simulink model "Antriebsstrangmodell_V1_4_n5_WHasym"  (R2019a)
settings: Solver=FixedStepAuto  StartTime=0.0  StopTime=t_Simulation  FixedStep=dt  RelTol=1e-3
values from neighbouring files (symbols this model uses):
  A_Stirn = 2    [Simulation_Antriebsstrangmodell_V1_4_n5_WHasym.m]    (also in Simulation_Antriebsstrangmodell_V1_4_n5_WHasym_S1.m)
  alpha_Luft = -4e-3    (= -0.004)    [Simulation_Antriebsstrangmodell_V1_4_n5_WHasym.m]    (also in Simulation_Antriebsstrangmodell_V1_4_n5_WHasym_S1.m)
  alpha_Rotor = alpha_Al    (= 0.004)    [Simulation_Antriebsstrangmodell_V1_4_n5_WHasym.m]    (also in Simulation_Antriebsstrangmodell_V1_4_n5_WHasym_S1.m)
  alpha_Stator = alpha_Al    (= 0.004)    [Simulation_Antriebsstrangmodell_V1_4_n5_WHasym.m]    (also in Simulation_Antriebsstrangmodell_V1_4_n5_WHasym_S1.m)
  alpha_Ummag = -0.75e-3    (= -0.00075)    [Simulation_Antriebsstrangmodell_V1_4_n5_WHasym.m]    (also in Simulation_Antriebsstrangmodell_V1_4_n5_WHasym_S1.m)
  c_W = 0.37    [Simulation_Antriebsstrangmodell_V1_4_n5_WHasym.m]    (also in Simulation_Antriebsstrangmodell_V1_4_n5_WHasym_S1.m)
  cp_Luft = 1008.8    [Simulation_Antriebsstrangmodell_V1_4_n5_WHasym.m]    (also in Simulation_Antriebsstrangmodell_V1_4_n5_WHasym_S1.m)
  e_Fahrzeug = 1.0478    [Simulation_Antriebsstrangmodell_V1_4_n5_WHasym.m]    (also in Simulation_Antriebsstrangmodell_V1_4_n5_WHasym_S1.m)
  eta_EMaschine_Break_M_EMaschine = flipud(KennfeldMaschine.M(:,1))'    [Simulation_Antriebsstrangmodell_V1_4_n5_WHasym.m]    (also in Simulation_Antriebsstrangmodell_V1_4_n5_WHasym_S1.m)
  eta_EMaschine_Break_M_EMaschine_reku = -KennfeldMaschine.M(:,1)'    [Simulation_Antriebsstrangmodell_V1_4_n5_WHasym.m]    (also in Simulation_Antriebsstrangmodell_V1_4_n5_WHasym_S1.m)
  eta_EMaschine_Break_n_EMaschine = KennfeldMaschine.n(end-1,:)    [Simulation_Antriebsstrangmodell_V1_4_n5_WHasym.m]    (also in Simulation_Antriebsstrangmodell_V1_4_n5_WHasym_S1.m)
  eta_EMaschine_Break_n_EMaschine_reku = KennfeldMaschine.n(end-1,:)    [Simulation_Antriebsstrangmodell_V1_4_n5_WHasym.m]    (also in Simulation_Antriebsstrangmodell_V1_4_n5_WHasym_S1.m)
  eta_EMaschine_Faktor_Volllast = 0.98    [Simulation_Antriebsstrangmodell_V1_4_n5_WHasym.m]    (also in Simulation_Antriebsstrangmodell_V1_4_n5_WHasym_S1.m)
  eta_EMaschine_Table = flip(KennfeldMaschine.etages,1)    [Simulation_Antriebsstrangmodell_V1_4_n5_WHasym.m]    (also in Simulation_Antriebsstrangmodell_V1_4_n5_WHasym_S1.m)
  eta_EMaschine_Table_reku = KennfeldMaschine.etages    [Simulation_Antriebsstrangmodell_V1_4_n5_WHasym.m]    (also in Simulation_Antriebsstrangmodell_V1_4_n5_WHasym_S1.m)
  eta_Getriebe = 0.96    [Simulation_Antriebsstrangmodell_V1_4_n5_WHasym.m]    (also in Simulation_Antriebsstrangmodell_V1_4_n5_WHasym_S1.m)
  eta_IA = 0.5    [Simulation_Antriebsstrangmodell_V1_4_n5_WHasym.m]    (also in Simulation_Antriebsstrangmodell_V1_4_n5_WHasym_S1.m)
  h_WC_pumpoff = Nu_WC*lam_WC/dh_WC    [Simulation_Antriebsstrangmodell_V1_4_n5_WHasym.m]    (also in Simulation_Antriebsstrangmodell_V1_4_n5_WHasym_S1.m)
  h_WC_pumpon = Nu_WC*lam_WC/dh_WC    [Simulation_Antriebsstrangmodell_V1_4_n5_WHasym.m]    (also in Simulation_Antriebsstrangmodell_V1_4_n5_WHasym_S1.m)
  i_Getriebe = 5.697    [Simulation_Antriebsstrangmodell_V1_4_n5_WHasym.m]    (also in Simulation_Antriebsstrangmodell_V1_4_n5_WHasym_S1.m)
  krb_Korrektur = 0.53/10    (= 0.053)    [Simulation_Antriebsstrangmodell_V1_4_n5_WHasym.m]    (also in Simulation_Antriebsstrangmodell_V1_4_n5_WHasym_S1.m)
  lam_Luft = 0.028592    [Simulation_Antriebsstrangmodell_V1_4_n5_WHasym.m]    (also in Simulation_Antriebsstrangmodell_V1_4_n5_WHasym_S1.m)
  M_EMaschine_max = zeros(2,numel(eta_EMaschine_Break_n_EMaschine))    [Simulation_Antriebsstrangmodell_V1_4_n5_WHasym.m]    (also in Simulation_Antriebsstrangmodell_V1_4_n5_WHasym_S1.m)
  m_Fahrzeug = 825    [Simulation_Antriebsstrangmodell_V1_4_n5_WHasym.m]    (also in Simulation_Antriebsstrangmodell_V1_4_n5_WHasym_S1.m)
  m_Zuladung = 80    [Simulation_Antriebsstrangmodell_V1_4_n5_WHasym.m]    (also in Simulation_Antriebsstrangmodell_V1_4_n5_WHasym_S1.m)
  nue_Luft = 19.230034390524e-6    (= 1.92300343905e-05)    [Simulation_Antriebsstrangmodell_V1_4_n5_WHasym.m]    (also in Simulation_Antriebsstrangmodell_V1_4_n5_WHasym_S1.m)
  pump_start_limit = 273.15 + 33    (= 306.15)    [Simulation_Antriebsstrangmodell_V1_4_n5_WHasym.m]    (also in Simulation_Antriebsstrangmodell_V1_4_n5_WHasym_S1.m)
  r_dynamisch = 0.2774    [Simulation_Antriebsstrangmodell_V1_4_n5_WHasym.m]    (also in Simulation_Antriebsstrangmodell_V1_4_n5_WHasym_S1.m)
  rho_Luft = 1.2    [Simulation_Antriebsstrangmodell_V1_4_n5_WHasym.m]    (also in Simulation_Antriebsstrangmodell_V1_4_n5_WHasym_S1.m)
  rho_Luft_EM = 1.0468    [Simulation_Antriebsstrangmodell_V1_4_n5_WHasym.m]    (also in Simulation_Antriebsstrangmodell_V1_4_n5_WHasym_S1.m)
  share_EMaschine_Ummagnet_reku_Table = ser.gen.share_Ummagnetisierungsverluste    [Simulation_Antriebsstrangmodell_V1_4_n5_WHasym.m]    (also in Simulation_Antriebsstrangmodell_V1_4_n5_WHasym_S1.m)
  share_EMaschine_Ummagnet_Table = ser.mot.share_Ummagnetisierungsverluste    [Simulation_Antriebsstrangmodell_V1_4_n5_WHasym.m]    (also in Simulation_Antriebsstrangmodell_V1_4_n5_WHasym_S1.m)
  share_EMaschine_Wicklung_reku_Table = ser.gen.share_Wicklungsverluste    [Simulation_Antriebsstrangmodell_V1_4_n5_WHasym.m]    (also in Simulation_Antriebsstrangmodell_V1_4_n5_WHasym_S1.m)
  share_EMaschine_Wicklung_Table = ser.mot.share_Wicklungsverluste    [Simulation_Antriebsstrangmodell_V1_4_n5_WHasym.m]    (also in Simulation_Antriebsstrangmodell_V1_4_n5_WHasym_S1.m)
  share_EMaschine_WirkMech_reku_Table = ser.gen.share_WirkmechVerluste    [Simulation_Antriebsstrangmodell_V1_4_n5_WHasym.m]    (also in Simulation_Antriebsstrangmodell_V1_4_n5_WHasym_S1.m)
  share_EMaschine_WirkMech_Table = ser.mot.share_WirkmechVerluste    [Simulation_Antriebsstrangmodell_V1_4_n5_WHasym.m]    (also in Simulation_Antriebsstrangmodell_V1_4_n5_WHasym_S1.m)
  share_EMaschine_WirkZus_reku_Table = ser.gen.share_WirkZusVerl    [Simulation_Antriebsstrangmodell_V1_4_n5_WHasym.m]    (also in Simulation_Antriebsstrangmodell_V1_4_n5_WHasym_S1.m)
  share_EMaschine_WirkZus_Table = ser.mot.share_WirkZusVerl    [Simulation_Antriebsstrangmodell_V1_4_n5_WHasym.m]    (also in Simulation_Antriebsstrangmodell_V1_4_n5_WHasym_S1.m)
  T_Entwurf_Rotor = 273.15+20    (= 293.15)    [Simulation_Antriebsstrangmodell_V1_4_n5_WHasym.m]    (also in Simulation_Antriebsstrangmodell_V1_4_n5_WHasym_S1.m)
  T_Entwurf_Stator = 273.15+20    (= 293.15)    [Simulation_Antriebsstrangmodell_V1_4_n5_WHasym.m]    (also in Simulation_Antriebsstrangmodell_V1_4_n5_WHasym_S1.m)
  t_Simulation = v_Fahrzeug.Time(end)+1    [Simulation_Antriebsstrangmodell_V1_4_n5_WHasym.m]    (also in Simulation_Antriebsstrangmodell_V1_4_n5_WHasym_S1.m = v_Fahrzeug.Time(end))
  T_Start_EMaschine = 273.15 + 23    (= 296.15)    [Simulation_Antriebsstrangmodell_V1_4_n5_WHasym.m]    (also in Simulation_Antriebsstrangmodell_V1_4_n5_WHasym_S1.m)
  v_max = 110    [Simulation_Antriebsstrangmodell_V1_4_n5_WHasym.m]    (also in Simulation_Antriebsstrangmodell_V1_4_n5_WHasym_S1.m)
undefined symbols (not defined in the file or in its folder): A_AGP, A_IA, Anteil_Rotor_Ringe, Anteil_Stator, chi_Lager, D_2a, D_2r, delta, f_R, m_RTO, m_RYO, m_SSL_L, m_STO, m_SYO, m_WH1_L, m_WH2_L, n_dis
libraries: fl_lib x440, nesl_utility x106, SimscapeCustomBlocks_lib x45, simulink x3
(part 5 of 5)

== system Antriebsstrangmodell_V1_4_n5_WHasym/Antriebsstrang/E-Maschine Thermik/Wärmeübergangskoeffizienten Konvektion Luftspalt und Endcap-Luft/Endcap-Luft-Konvektion ==
  note: HTC_fconv stellt den Wärmeübergangs-
      | koeffizienten der erzwungen dar. Für diesen
      | wird bloß der geschwindigkeitsabhängige
      | Teil der empirischen Konvektions-Korrelation
      | der Innenluft genommen.
  note: Zusammenhang zwischen Geschwindigkeit der Innenluft und dem konvektiven Wärmeübergangskoeffizienten nach MELLOR 1991.
      | eta_IA ist hierbei der Lüfterwirkungsgrad, der das Verhältnis von Innenluftgeschwindigkeit zur Umfangsgeschwindigkeit des Kurzschlussrings am Rotor darstellt.
  n_EMaschine [min^-1] : Inport
  Add1 : Sum
  Constant1 : Constant  Value=0.29
  Constant2 : Constant
  Constant3 : Constant  Value=15.5
  Constant4 : Constant  Value=eta_IA
  Constant6 : Constant  Value=D_2r
  Divide1 : Product  Inputs=**
  Divide2 : Product  Inputs=**
  Divide3 : Product  Inputs=***
  Divide4 : Product  Inputs=**
  Gain : Gain  Gain=2*pi/60
  Gain1 : Gain  Gain=0.5
  HTC_Innenluft [W*m^-2*K^-1] : Outport
  HTC_fconv_Innenluft [W*m^-2*K^-1] : Outport  Port=2
  wires:
  Divide3/1 -> Divide1/1  "v_IA Innenluftgeschwindigkeit [m*s^-1]"
  n_EMaschine [min^-1]/1 -> Gain/1
  Constant6/1 -> Gain1/1
  Gain/1 -> Divide3/1
  Constant4/1 -> Divide3/2
  Gain1/1 -> Divide3/3
  Constant1/1 -> Divide1/2
  Divide1/1 -> Divide4/1, Add1/1
  Constant2/1 -> Add1/2
  Add1/1 -> Divide2/1
  Constant3/1 -> Divide4/2, Divide2/2
  Divide2/1 -> HTC_Innenluft [W*m^-2*K^-1]/1
  Divide4/1 -> HTC_fconv_Innenluft [W*m^-2*K^-1]/1

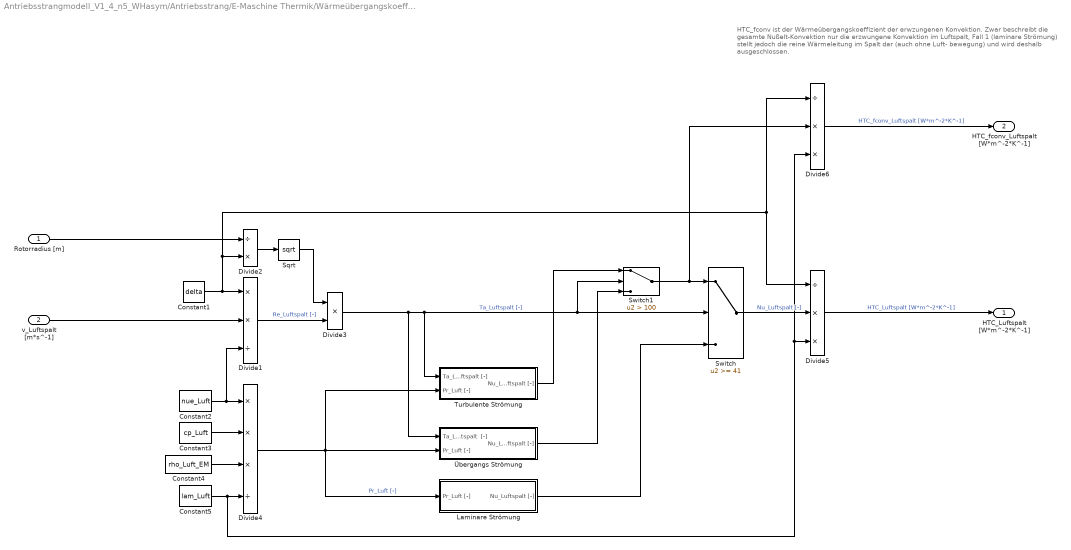
== system Antriebsstrangmodell_V1_4_n5_WHasym/Antriebsstrang/E-Maschine Thermik/Wärmeübergangskoeffizienten Konvektion Luftspalt und Endcap-Luft/Luftspalt-Konvektion ==
  note: HTC_fconv ist der Wärmeübergangskoeffizient der erwzungenen Konvektion.
      | Zwar beschreibt die gesamte Nußelt-Konvektion nur die erzwungene Konvektion im Luftspalt,
      | Fall 1 (laminare Strömung) stellt jedoch die reine Wärmeleitung im Spalt dar (auch ohne Luft-
      | bewegung) und wird deshalb ausgeschlossen.
  Rotorradius [m] : Inport
  v_Luftspalt [m*s^-1] : Inport  Port=2
  Constant1 : Constant  Value=delta
  Constant2 : Constant  Value=nue_Luft
  Constant3 : Constant  Value=cp_Luft
  Constant4 : Constant  Value=rho_Luft_EM
  Constant5 : Constant  Value=lam_Luft
  Divide1 : Product  Inputs=**/
  Divide2 : Product  Inputs=/*
  Divide3 : Product  Inputs=**
  Divide4 : Product  Inputs=***/
  Divide5 : Product  Inputs=/**
  Divide6 : Product  Inputs=/**
  Laminare Strömung : Subsystem
  Sqrt : Sqrt  SaturateOnIntegerOverflow=on
  Switch : Switch  Threshold=41
  Switch1 : Switch  Criteria=u2 > Threshold  Threshold=100
  Turbulente Strömung : Subsystem
  Übergangs Strömung : Subsystem
  HTC_Luftspalt [W*m^-2*K^-1] : Outport
  HTC_fconv_Luftspalt [W*m^-2*K^-1] : Outport  Port=2
  wires:
  Divide3/1 -> Switch1/2, Switch/2, Turbulente Strömung/1(Ta_Luftspalt [-]), Übergangs Strömung/1(Ta_Luftspalt  [-])  "Ta_Luftspalt [-]"
  Constant4/1 -> Divide4/3
  Divide4/1 -> Übergangs Strömung/2(Pr_Luft [-]), Laminare Strömung/1(Pr_Luft [-]), Turbulente Strömung/2(Pr_Luft [-])  "Pr_Luft [-]"
  Rotorradius [m]/1 -> Divide2/1
  Constant2/1 -> Divide1/3, Divide4/1
  Laminare Strömung/1(Nu_Luftspalt [-]) -> Switch/3
  Turbulente Strömung/1(Nu_Luftspalt [-]) -> Switch1/1
  Constant1/1 -> Divide6/1, Divide5/1, Divide2/2, Divide1/1
  Übergangs Strömung/1(Nu_Luftspalt [-]) -> Switch1/3
  Constant5/1 -> Divide6/3, Divide5/3, Divide4/4
  Divide1/1 -> Divide3/2  "Re_Luftspalt [-]"
  Switch1/1 -> Divide6/2, Switch/1
  Switch/1 -> Divide5/2  "Nu_Luftspalt [-]"
  Sqrt/1 -> Divide3/1
  v_Luftspalt [m*s^-1]/1 -> Divide1/2
  Divide5/1 -> HTC_Luftspalt [W*m^-2*K^-1]/1  "HTC_Luftspalt [W*m^-2*K^-1]"
  Constant3/1 -> Divide4/2
  Divide2/1 -> Sqrt/1
  Divide6/1 -> HTC_fconv_Luftspalt [W*m^-2*K^-1]/1  "HTC_fconv_Luftspalt [W*m^-2*K^-1]"

== system Antriebsstrangmodell_V1_4_n5_WHasym/Antriebsstrang/E-Maschine Verlustleistung/Wikrungsgrad und Verlustleistung - Antrieb/Korrektur der Gesamt-Verlustleistung ==
  P_EMaschine_Verlust [W] : Inport
  M_EMaschine_ist [Nm] : Inport  Port=2
  n_EMaschine [min^-1] : Inport  Port=3
  Anteil WirkMechVerluste Antrieb : Lookup_n-D  BreakpointsForDimension1=eta_EMaschine_Break_M_EMaschine  BreakpointsForDimension2=eta_EMaschine_Break_n_EMaschine  BeginIndexSearchUsingPreviousIndexResult=on  Table=share_EMaschine_WirkMech_Table  ExtrapMethod=Clip  UseLastTableValue=on  InternalRulePriority=Speed  RndMeth=Simplest  InputSameDT=on
  Constant : Constant
  Constant1 : Constant  Value=krb_Korrektur
  Constant2 : Constant
  Divide1 : Product  Inputs=**
  Divide2 : Product  Inputs=**
  Sum : Sum  Inputs=+-
  Sum1 : Sum  Inputs=+-
  P_EMaschine_Verlust_korr [W] : Outport
  wires:
  P_EMaschine_Verlust [W]/1 -> Divide2/1
  n_EMaschine [min^-1]/1 -> Anteil WirkMechVerluste Antrieb/2
  M_EMaschine_ist [Nm]/1 -> Anteil WirkMechVerluste Antrieb/1
  Divide2/1 -> P_EMaschine_Verlust_korr [W]/1  "P_EMaschine_Verlust_korr [W]"
  Constant/1 -> Sum/1
  Constant1/1 -> Sum/2
  Sum/1 -> Divide1/2
  Anteil WirkMechVerluste Antrieb/1 -> Divide1/1  "Anteil_WirkMechVerluste [-]"
  Constant2/1 -> Sum1/1
  Divide1/1 -> Sum1/2
  Sum1/1 -> Divide2/2

== system Antriebsstrangmodell_V1_4_n5_WHasym/Antriebsstrang/E-Maschine Verlustleistung/Wikrungsgrad und Verlustleistung - Rekuperation/Korrektur der Gesamt-Verlustleistung ==
  P_EMaschine_Verlust [W] : Inport
  M_EMaschine_ist [Nm] : Inport  Port=2
  n_EMaschine [min^-1] : Inport  Port=3
  Abs : Abs
  Anteil WirkMechVerluste Reku : Lookup_n-D  BreakpointsForDimension1=eta_EMaschine_Break_M_EMaschine  BreakpointsForDimension2=eta_EMaschine_Break_n_EMaschine  BeginIndexSearchUsingPreviousIndexResult=on  Table=share_EMaschine_WirkMech_reku_Table  ExtrapMethod=Clip  UseLastTableValue=on  InternalRulePriority=Speed  RndMeth=Simplest  InputSameDT=on
  Constant : Constant
  Constant1 : Constant  Value=krb_Korrektur
  Constant2 : Constant
  Divide1 : Product  Inputs=**
  Divide2 : Product  Inputs=**
  Scope : Scope
  Sum : Sum  Inputs=+-
  Sum1 : Sum  Inputs=+-
  P_EMaschine_Verlust_korr [W] : Outport
  wires:
  P_EMaschine_Verlust [W]/1 -> Divide2/1
  n_EMaschine [min^-1]/1 -> Anteil WirkMechVerluste Reku/2
  M_EMaschine_ist [Nm]/1 -> Abs/1
  Divide2/1 -> P_EMaschine_Verlust_korr [W]/1  "P_EMaschine_Verlust_korr [W]"
  Constant/1 -> Sum/1
  Constant1/1 -> Sum/2
  Sum/1 -> Divide1/2
  Anteil WirkMechVerluste Reku/1 -> Scope/1, Divide1/1  "Anteil_WirkMechVerluste [-]"
  Constant2/1 -> Sum1/1
  Divide1/1 -> Sum1/2
  Sum1/1 -> Divide2/2
  Abs/1 -> Anteil WirkMechVerluste Reku/1

== system Antriebsstrangmodell_V1_4_n5_WHasym/Antriebsstrang/E-Maschine Thermik/Wärmeübergangskoeffizienten Konvektion Luftspalt und Endcap-Luft/Luftspalt-Konvektion/Laminare Strömung ==
  Pr_Luft [-] : Inport
  Constant6 : Constant  Value=41
  Constant7 : Constant  Value=0.63
  Constant8 : Constant  Value=0.202
  Constant9 : Constant  Value=0.27
  Divide5 : Product  Inputs=***
  Math Function : Math  Operator=pow  SaturateOnIntegerOverflow=on
  Math Function1 : Math  Operator=pow  SaturateOnIntegerOverflow=on
  Nu_Luftspalt [-] : Outport
  wires:
  Constant6/1 -> Math Function/1
  Constant7/1 -> Math Function/2
  Math Function/1 -> Divide5/2
  Math Function1/1 -> Divide5/3
  Constant9/1 -> Math Function1/2
  Pr_Luft [-]/1 -> Math Function1/1
  Constant8/1 -> Divide5/1
  Divide5/1 -> Nu_Luftspalt [-]/1  "Nu_Luftspalt [-]"

== system Antriebsstrangmodell_V1_4_n5_WHasym/Antriebsstrang/E-Maschine Thermik/Wärmeübergangskoeffizienten Konvektion Luftspalt und Endcap-Luft/Luftspalt-Konvektion/Turbulente Strömung ==
  Ta_Luftspalt [-] : Inport
  Pr_Luft [-] : Inport  Port=2
  Constant7 : Constant  Value=0.5
  Constant8 : Constant  Value=0.386
  Constant9 : Constant  Value=0.27
  Divide5 : Product  Inputs=***
  Math Function : Math  Operator=pow  SaturateOnIntegerOverflow=on
  Math Function1 : Math  Operator=pow  SaturateOnIntegerOverflow=on
  Nu_Luftspalt [-] : Outport
  wires:
  Ta_Luftspalt [-]/1 -> Math Function/1
  Constant7/1 -> Math Function/2
  Math Function/1 -> Divide5/2
  Math Function1/1 -> Divide5/3
  Constant9/1 -> Math Function1/2
  Pr_Luft [-]/1 -> Math Function1/1
  Constant8/1 -> Divide5/1
  Divide5/1 -> Nu_Luftspalt [-]/1  "Nu_Luftspalt [-]"

== system Antriebsstrangmodell_V1_4_n5_WHasym/Antriebsstrang/E-Maschine Thermik/Wärmeübergangskoeffizienten Konvektion Luftspalt und Endcap-Luft/Luftspalt-Konvektion/Übergangs Strömung ==
  Ta_Luftspalt  [-] : Inport
  Pr_Luft [-] : Inport  Port=2
  Constant7 : Constant  Value=0.63
  Constant8 : Constant  Value=0.202
  Constant9 : Constant  Value=0.27
  Divide5 : Product  Inputs=***
  Math Function : Math  Operator=pow  SaturateOnIntegerOverflow=on
  Math Function1 : Math  Operator=pow  SaturateOnIntegerOverflow=on
  Nu_Luftspalt [-] : Outport
  wires:
  Ta_Luftspalt  [-]/1 -> Math Function/1
  Constant7/1 -> Math Function/2
  Math Function/1 -> Divide5/2
  Math Function1/1 -> Divide5/3
  Constant9/1 -> Math Function1/2
  Pr_Luft [-]/1 -> Math Function1/1
  Constant8/1 -> Divide5/1
  Divide5/1 -> Nu_Luftspalt [-]/1  "Nu_Luftspalt [-]"
